simulink model "F1_Telemetry_Sim"  (R2025a)
settings: Solver=VariableStepAuto  StartTime=0.0  StopTime=10.0  RelTol=1e-3
undefined symbols (not defined in the file or in its folder): canChannel
libraries: canlib x2
settings Model: Creator=sunda  LastModifiedBy=sunda

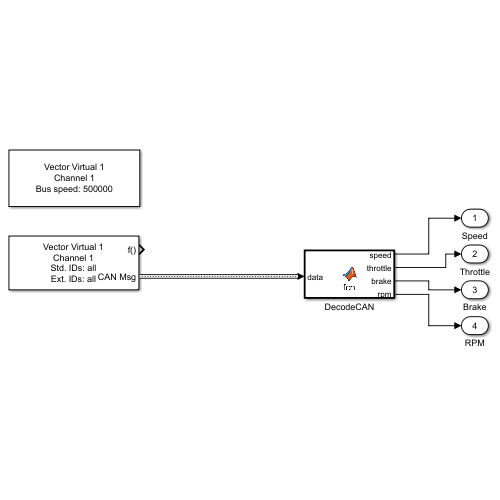
[thumbnail: Simulink's stored preview of the top-level diagram]
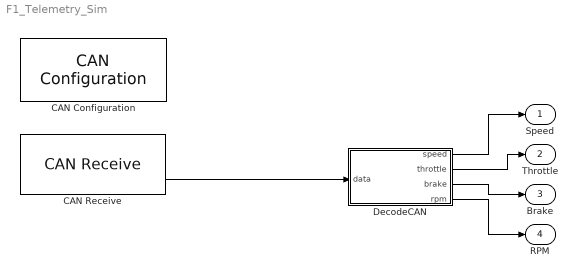
== system F1_Telemetry_Sim ==
  CAN Configuration : canlib/CAN Configuration  BlockHandle=158.0005  Device=Vector Virtual 1 (Channel 1)  DeviceMenu=Vector Virtual 1 (Channel 1)  ObjConstructor=canChannel('Vector', 'Virtual 1', 1)  BusSpeed=500000  EnableBitParameters=off  SJW=1  TSEG1=10  TSEG2=5  NSamples=1  AckMode=Normal
  CAN Receive : canlib/CAN Receive  BlockHandle=163.0005  Device=Vector Virtual 1 (Channel 1)  DeviceMenu=Vector Virtual 1 (Channel 1)  ObjConstructor=canChannel('Vector', 'Virtual 1', 1)  EnableStandardIDsFilter=off  StdIDsCombo=Allow all  StandardIDs=0  EnableExtendedIDsFilter=off  ExtIDsCombo=Allow all  ExtendedIDs=0  SampleTime=0.01  MsgsPerTimestep=all  InternalFilterUpdateStatus=on  BusOutput=on
  DecodeCAN : MATLAB Function  TreatAsAtomicUnit=on
  Speed : Outport
  Throttle : Outport  Port=2
  Brake : Outport  Port=3
  RPM : Outport  Port=4
  wires:
  DecodeCAN/1(speed) -> Speed/1
  DecodeCAN/2(throttle) -> Throttle/1
  DecodeCAN/3(brake) -> Brake/1
  DecodeCAN/4(rpm) -> RPM/1
  CAN Receive/2 -> DecodeCAN/1(data)

== matlab function F1_Telemetry_Sim/DecodeCAN ==
  data: data input; speed output; throttle output; brake output; rpm output
function [speed, throttle, brake, rpm] = fcn(data)
    %#codegen
    % Assume data is a uint8 vector of length >= 6
    % Add a check to avoid out-of-bounds error during model compilation
    if length(data) < 6
        speed = 0;
        throttle = 0;
        brake = 0;
        rpm = 0;
    else
        speed = double(data(1));
        throttle = double(data(2));
        brake = double(data(3));
        rpm = double(bitshift(data(5), 8) + data(6));
    end
end
